simulink model "ex04_laptop"  (R2020b)
settings: Solver=VariableStepAuto  StartTime=0.0  StopTime=60  RelTol=1e-3
model workspace (MAT data in the model file):
  courseObject.course = 'stateflow'
  courseObject.chapter = 3
  courseObject.lesson = 3
  courseObject.section = 1
  courseObject.task = 1
undefined symbols (not defined in the file): sigbuilder_block
settings Model: EnablePacing=on  PacingRate=3  Creator=gb  LastModifiedBy=19255551
settings DataIOCC: SaveTime=off

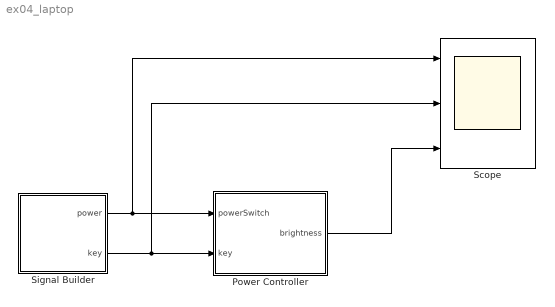
== system ex04_laptop ==
  Power Controller : Stateflow chart  TreatAsAtomicUnit=on
  Scope : Scope  NumInputPorts=3
  Signal Builder : Subsystem  Tag=STV Subsys  LoadFcn=sigbuilder_block('load');  StartFcn=sigbuilder_block('start');  StopFcn=sigbuilder_block('stop');  ClipboardFcn=sigbuilder_block('clipboard');  mask(Sigbuilder block){tuvar=[0:10]}
      mask help: Simulink:masks:SigbuilderBlock_MD
      mask init:
      | if ~strcmp(get_param(bdroot(gcbh),'SimulationStatus'),'stopped') tuvar = sigbuilder_block('maskInit'); end
      settings: CopyFcn=sigbuilder_block('copy');  DeleteFcn=sigbuilder_block('delete');  ModelCloseFcn=sigbuilder_block('modelClose');  PreSaveFcn=sigbuilder_block('preSave');  PauseFcn=sigbuilder_block('pause');  ContinueFcn=sigbuilder_block('continue');  NameChangeFcn=sigbuilder_block('namechange');  OpenFcn=sigbuilder_block('open',[4.8 22.8 1142.4 538.8 ]);  CloseFcn=sigbuilder_block('close');
      mask Display: plot(0, 0, 100, 100,[2, 2, 32, 32, 2], [68, 8, 8, 68, 68],[32, 2], [38, 38], [32, 19, 2],[53, 60, 44], [32, 17, 17, 2],[16, 16, 31, 31]);txt = getActiveGroup(gcbh);text(2, 100, txt,'verticalAlignment', 'top');
  wires:
  Signal Builder/1(power) -> Scope/1, Power Controller/1(powerSwitch)
  Signal Builder/2(key) -> Scope/2, Power Controller/2(key)
  Power Controller/1(brightness) -> Scope/3

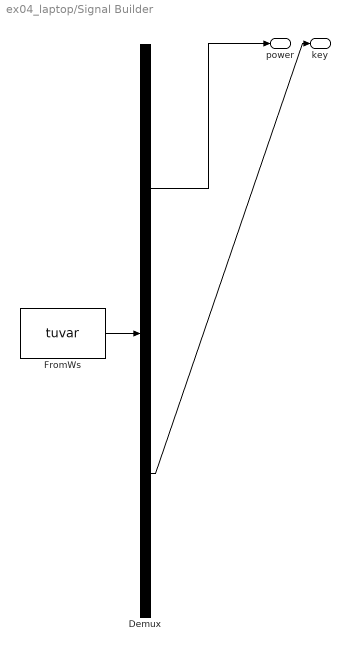
== system ex04_laptop/Signal Builder ==
  Demux : Demux  Tag=STV Demux  Outputs=2
      settings: DisplayOption=none
  FromWs : FromWorkspace  Tag=STV FromWs  VariableName=tuvar
      SigBuilderData=|
      | common.afterFinalStr = 'Extrapolate'
      | common.sampleTime = 0
      | dataSet.timeRange = [0 60]
      | dataSet.name = 'Group 1'
      | sbobj.Groups.Name = 'Group 1'
      | sbobj.Groups.Signals(1).Name = 'power'
      | sbobj.Groups.Signals(1).XData = [0 2 2 36 36 40 40 59 59 60]
      | sbobj.Groups.Signals(1).YData = [0 0 1 1 0 0 1 1 0 0]
      | sbobj.Groups.Signals(2).Name = 'key'
      | sbobj.Groups.Signals(2).XData = [0 10 10 11 11 20 20 21 21 25 25 26 26 37 37 38 38 42 42 43 43 44 44 45 45 46 46 47 47 48 48 49 49 50 50 51 51 60]
      | sbobj.Groups.Signals(2).YData = [0 0 1 1 0 0 1 1 0 0 1 1 0 0 1 1 0 0 1 1 0 0 1 1 0 0 1 1 0 0 1 1 0 0 1 1 0 0]
      | sbobj.Groups.TimeRange = [0 60]
  power : Outport  Tag=STV Outport
  key : Outport  Tag=STV Outport  Port=2
  wires:
  Demux/1 -> power/1
  FromWs/1 -> Demux/1
  Demux/2 -> key/1

== stateflow chart ex04_laptop/Power Controller ==
  state laptop
    state machineOff
      entry:
      brightness = 0;
    state mahinceOn
      state fullBrightness
        entry:
        brightness = 1;
      state halfBrightness
        entry:
        brightness = 0.5
      state screenOff
        entry:
        brightness = 0;
      (default) -> fullBrightness
      fullBrightness -> halfBrightness : after(3,sec)
      halfBrightness -> fullBrightness [order 2] : [key == 1]
      screenOff -> fullBrightness : [key == 1]
      halfBrightness -> screenOff [order 1] : after(3,sec)
    (default) -> machineOff
    machineOff -> mahinceOn : [powerSwitch == 1]
    mahinceOn -> machineOff : [powerSwitch == 0]
  (default) -> laptop
  data: powerSwitch input; key input; brightness output
